simulink model "Ex2s"  (R2025a)
settings: Solver=VariableStepAuto  StartTime=0.0  StopTime=40  RelTol=1e-3
undefined symbols (not defined in the file): A, B, C, C_2, D, D_2, fi_1, gama_1

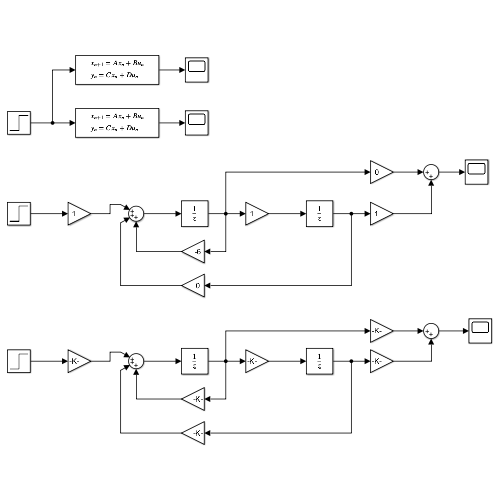
[thumbnail: Simulink's stored preview of the top-level diagram]
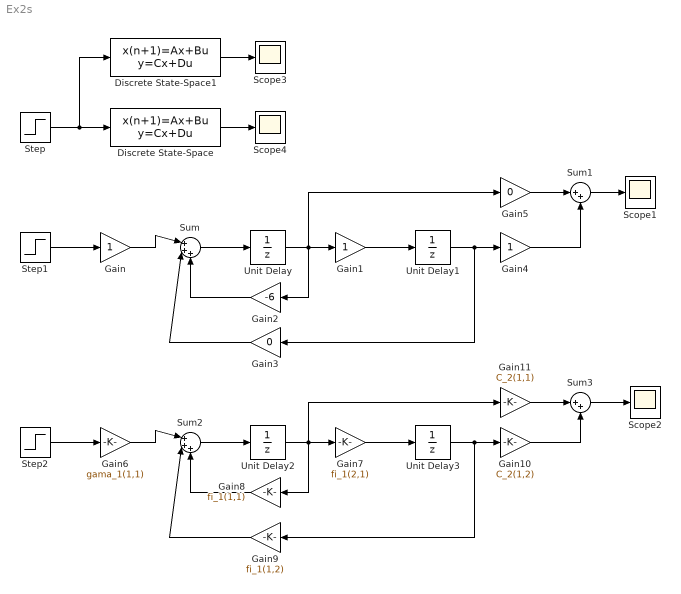
== system Ex2s ==
  Discrete State-Space : DiscreteStateSpace  A=fi_1  B=gama_1  C=C_2  D=D_2  SampleTime=-1
  Discrete State-Space1 : DiscreteStateSpace  A=A  B=B  C=C  D=D  SampleTime=-1
  Gain : Gain
  Gain1 : Gain
  Gain10 : Gain  Gain=C_2(1,2)
  Gain11 : Gain  Gain=C_2(1,1)
  Gain2 : Gain  Gain=-6
  Gain3 : Gain  Gain=0
  Gain4 : Gain
  Gain5 : Gain  Gain=0
  Gain6 : Gain  Gain=gama_1(1,1)
  Gain7 : Gain  Gain=fi_1(2,1)
  Gain8 : Gain  Gain=fi_1(1,1)
  Gain9 : Gain  Gain=fi_1(1,2)
  Scope{1..4} (4 alike) : Scope
      Scope1 settings: ActiveDisplayYMinimum=-6.0781431848247783E+28  ActiveDisplayYMaximum=1.6576754140431214E+28
      Scope2 settings: ActiveDisplayYMinimum=-0.12508732625482455  ActiveDisplayYMaximum=1.1257859362934213  DataLoggingVariableName=ScopeData2
      Scope3 settings: ActiveDisplayYMinimum=-6.0781431848247783E+28  ActiveDisplayYMaximum=1.6576754140431214E+28
      Scope4 settings: ActiveDisplayYMinimum=-6.0781431848247783E+28  ActiveDisplayYMaximum=1.6576754140431214E+28  DataLoggingVariableName=ScopeData3
  Step : Step  SampleTime=1
  Step1 : Step  SampleTime=1
  Step2 : Step  SampleTime=1
  Sum : Sum  Inputs=|+++
  Sum1 : Sum  Inputs=|++
  Sum2 : Sum  Inputs=|+++
  Sum3 : Sum  Inputs=|++
  Unit Delay{,1..3} (4 alike) : UnitDelay  SampleTime=-1  HasFrameUpgradeWarning=on
  wires:
  Step/1 -> Discrete State-Space1/1, Discrete State-Space/1
  Step1/1 -> Gain/1
  Gain/1 -> Sum/1
  Sum/1 -> Unit Delay/1
  Unit Delay/1 -> Gain5/1, Gain2/1, Gain1/1
  Gain1/1 -> Unit Delay1/1
  Gain2/1 -> Sum/3
  Unit Delay1/1 -> Gain3/1, Gain4/1
  Gain3/1 -> Sum/2
  Gain5/1 -> Sum1/1
  Gain4/1 -> Sum1/2
  Sum1/1 -> Scope1/1
  Unit Delay2/1 -> Gain11/1, Gain7/1, Gain8/1
  Gain9/1 -> Sum2/2
  Unit Delay3/1 -> Gain9/1, Gain10/1
  Gain8/1 -> Sum2/3
  Gain7/1 -> Unit Delay3/1
  Sum2/1 -> Unit Delay2/1
  Gain6/1 -> Sum2/1
  Step2/1 -> Gain6/1
  Gain11/1 -> Sum3/1
  Gain10/1 -> Sum3/2
  Sum3/1 -> Scope2/1
  Discrete State-Space/1 -> Scope4/1
  Discrete State-Space1/1 -> Scope3/1
